simulink model "fulltry"  (R2023b)
settings: Solver=VariableStepAuto  StartTime=0.0  StopTime=40  RelTol=1e-3
undefined symbols (not defined in the file): C_dc, c_drt, C_p_opt, H_gen, H_vsm, H_WTR, I_dc_0, I_dc_base, Ibase_lv, k_d_vsm, k_drt, k_p_p_vsm, k_p_q_vsm, K_pitch, ki_q, L_d, l_f, L_grid, L_q, lambda_opt, Lbase1v, omega_nom, omega_WTR_min, omega_WTR_n, omega_WTR_sl, phase_shift_test_state, phase_shifts, pitch_max, pitch_min, Pitchanglevector, Pmax, Powercoefficient, psi_pm, R_a, r_f, R_grid, R_WTR, rate_max, rate_min, rocof_slope, Rocof_test_state, Sbase1, T_base, T_pitch, T_servo, Tchange_gfm_ref, Trocof_end, Trocof_start, Ts, TSRvector, V_dc, V_dc_base, v_w_n, Vbase_lv, voltage_sag_test_state, wind_array_step, Zbase1v
libraries: spsControlledVoltageSourceLib x6, spsPower3phInstantaneousLib x4, slpidlib x3, spsThreePhaseVIMeasurementLib x3, spsRMSLib x3, spsdq0toabcLib x2, spsCurrentMeasurementLib x2, spsSeriesRLCBranchLib x2, spsVoltageMeasurementLib x2, spsThreePhaseSeriesRLCBranchLib x2, spsDCVoltageSourceLib x2, spsGroundLib x1
(part 1 of 2)
settings Model: Creator=s183702  LastModifiedBy=marti

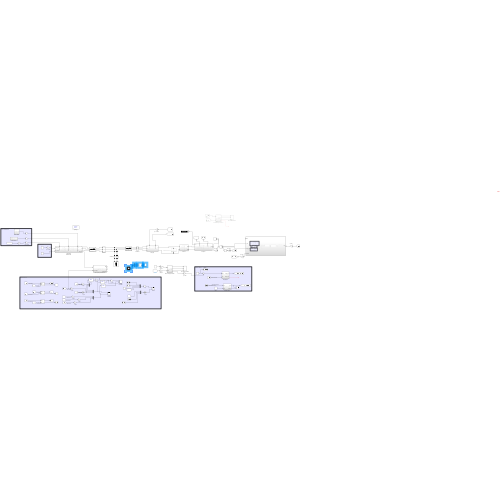
[thumbnail: Simulink's stored preview of the top-level diagram]
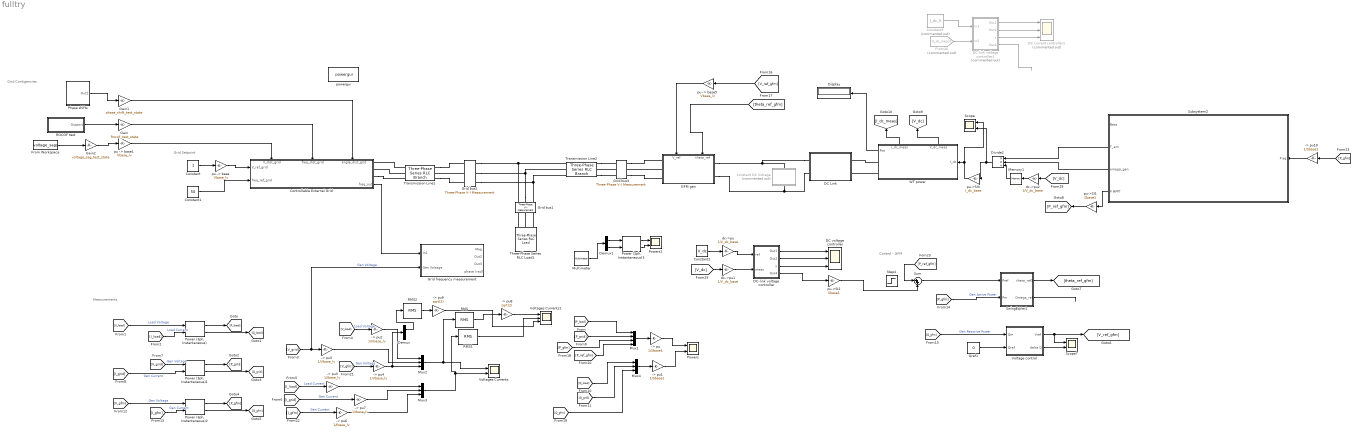
== system fulltry ==
  note: Control - GFM
  note: Grid Setpoint
  note: Grid Contigencies
  note: Measurements
  -> pu : Gain  Gain=1/Sbase1
  -> pu1 : Gain  Gain=1/Sbase1
  -> pu10 : Gain  Gain=1/Sbase1
  -> pu2 : Gain  Gain=1/Vbase_lv
  -> pu3 : Gain  Gain=1/Ibase_lv
  -> pu4 : Gain  Gain=1/Vbase_lv
  -> pu5 : Gain  Gain=1/Vbase_lv
  -> pu6 : Gain  Gain=1/Ibase_lv
  -> pu7 : Gain  Gain=1/Ibase_lv
  -> pu8 : Gain  Gain=sqrt(2)
  -> pu9 : Gain  Gain=sqrt(2)
  Constant : Constant
  Constant1 : Constant  Value=50
  Constant2 : Constant  Value=V_dc
  Constant3 : Constant  Commented=on  Value=I_dc_0
  Controllable External Grid : Subsystem
      settings: PortSchema="{\"entries\":[{\"content\":{\"sides\":[{\"content\":{\"connectorIds\":[\"In1\",\"In2\"]},\"type\":\"ConnectorPlacement.EquallySpacedRectSide\",\"uuid\":\"c82e3ee4-47de-4631-9682-a189e406d2fd\"},{\"content\":{\"connectorIds\":[\"RConn1\",\"RConn2\",\"RConn3\",\"Out1\"],\"side\":\"RIGHT\"},\"type\":\"ConnectorPlacement.EquallySpacedRectSide\",\"uuid\":\"b806e225-811d-4112-8c3d-45e9b8086e84\"},{\"content\":{\"connectorIds\":[\"In3\",\"In4\",\"In5\"],\"side\":\"TOP\"},\"type\":\"ConnectorPlacement.EquallySpacedRectSide\",\"uuid\":\"c79b677b-bc74-4454-b0f0-10f0f27e0767\"}]},\"type\":\"ConnectorPlacement.EquallySpacedConnector\",\"uuid\":\"44354c03-b4f0-403a-803b-b669dc1296a6\"}],\"packageUris\":[\"http://schema.mathworks.com/mf0/Connector/R2020b\"],\"version\":\"1.0\"}"
  DC Link : Subsystem
  DC current controller1 : Scope  Commented=on  NumInputPorts=3
  DC voltage controller : Scope  NumInputPorts=3
  DC-link voltage controller : Subsystem
  DC-link voltage controller1 : Subsystem  Commented=on
  Demux : Demux  Outputs=3
  Demux1 : Demux  Outputs=2
  Display : Display
  Divide2 : Product  Inputs=**/
  From Workspace : FromWorkspace  VariableName=voltage_sags
  From26 : From  Commented=on  GotoTag=I_dc_meas
  GFM gen : Subsystem
      settings: PortSchema="{\"entries\":[{\"content\":{\"sides\":[{\"content\":{\"connectorIds\":[\"LConn1\",\"LConn2\"]},\"type\":\"ConnectorPlacement.EquallySpacedRectSide\",\"uuid\":\"b9b898d8-aa2c-4fc0-879f-33950e845205\"},{\"content\":{\"connectorIds\":[\"RConn1\",\"RConn2\",\"RConn3\"],\"side\":\"RIGHT\"},\"type\":\"ConnectorPlacement.EquallySpacedRectSide\",\"uuid\":\"0f5f2870-ceda-40eb-961f-274893a00dd5\"},{\"content\":{\"connectorIds\":[\"In1\",\"In2\"],\"side\":\"TOP\"},\"type\":\"ConnectorPlacement.EquallySpacedRectSide\",\"uuid\":\"16b0f3cd-2bcf-4c98-bcc9-1e9131637ccf\"}]},\"type\":\"ConnectorPlacement.EquallySpacedConnector\",\"uuid\":\"5f5ec50b-7fca-4ced-b434-e49ba9676af4\"}],\"packageUris\":[\"http://schema.mathworks.com/mf0/Connector/R2020b\"],\"version\":\"1.0\"}"
  Gain : Gain  Gain=Rocof_test_state
  Gain1 : Gain  Gain=phase_shift_test_state
  Gain2 : Gain  Gain=voltage_sag_test_state
  Grid bus1 : spsThreePhaseVIMeasurementLib/Three-Phase V-I Measurement  VoltageMeasurement=phase-to-ground  SetLabelV=on  LabelV=V_load  Vpu=off  VpuLL=off  CurrentMeasurement=yes  SetLabelI=on  LabelI=I_load  Ipu=off  Pbase=100e6  Vbase=500e3  OutputType=Complex  PhasorSimulation=off  PSBequivalent=0
  Grid bus2 : spsThreePhaseVIMeasurementLib/Three-Phase V-I Measurement  VoltageMeasurement=phase-to-ground  SetLabelV=on  LabelV=V_grid  Vpu=off  VpuLL=off  CurrentMeasurement=yes  SetLabelI=on  LabelI=I_grid  Ipu=off  Pbase=100e6  Vbase=500e3  OutputType=Complex  PhasorSimulation=off  PSBequivalent=0
  Grid bus3 : spsThreePhaseVIMeasurementLib/Three-Phase V-I Measurement  VoltageMeasurement=phase-to-ground  SetLabelV=on  LabelV=V_gfm  Vpu=off  VpuLL=off  CurrentMeasurement=yes  SetLabelI=on  LabelI=I_gfm  Ipu=off  Pbase=100e6  Vbase=500e3  OutputType=Complex  PhasorSimulation=off  PSBequivalent=0
  Grid frequency measurement : Subsystem
  Memory1 : Memory  InitialCondition=V_dc
  Multimeter : spsMultimeterLib/Multimeter  L=6  sel=[1 2 3 4 5 6]  yselected={}  Gain=[1 1 1 1 1 1]  OutputType=Complex  PlotAtSimulationStop=off  PhasorSimulation=off
  Mux1 : Mux
  Mux2 : Mux  Inputs=3
  Mux3 : Mux  Inputs=3
  Mux4 : Mux  Inputs=3
  Phase shifts : Subsystem
  Power (3ph, Instantaneous){,1..3} (4 alike) : spsPower3phInstantaneousLib/Power (3ph, Instantaneous)
  Powers : Scope  NumInputPorts=2
  Powers1 : Scope  NumInputPorts=2
  Qref1 : Constant  Value=0
  RMS : spsRMSLib/RMS  TrueRMS=off  Freq=50  RMSInit=1  Ts=0
  RMS1 : spsRMSLib/RMS  TrueRMS=off  Freq=50  RMSInit=1  Ts=0
  RMS2 : spsRMSLib/RMS  TrueRMS=off  Freq=50  RMSInit=1  Ts=0
  ROCOF test : Subsystem
  Scope : Scope  NumInputPorts=2
  Scope7 : Scope  NumInputPorts=2
  Step4 : Step  Time=Tchange_gfm_ref  Before=Sbase1  After=Sbase1  SampleTime=0
  Subsystem2 : Subsystem
  Sum : Sum  Inputs=|++
  SwingEqVer1 : Subsystem
  Three-Phase Series RLC Load1 : spsThreePhaseSeriesRLCLoadLib/Three-Phase Series RLC Load  LConnTagsString=A|B|C  Configuration=Y (grounded)  NominalVoltage=Vbase_lv*sqrt(3/2)  Vabc=[1e3 1e3 1e3]  Vabcp=[1e3 1e3 1e3]  NominalFrequency=f_nom  UnbalancedPower=off  ActivePower=Sbase1*0.2  InductivePower=0  CapacitivePower=0  Pabc=[10e3 9e3 11e3]  QLabc=[100 90 110]  QCabc=[100 90 110]  Pabcp=[10e3 9e3 11e3]  QLabcp=[100 90 110]  QCabcp=[100 90 110]  Measurements=Branch voltages and currents  LoadType=constant PQ
  Transmission Line1 : spsThreePhaseSeriesRLCBranchLib/Three-Phase Series RLC Branch  LConnTagsString=A|B|C  RConnTagsString=A|B|C  BranchType=RL  Resistance=R_grid  Inductance=L_grid  Capacitance=0  Measurements=None
  Transmission Line2 : spsThreePhaseSeriesRLCBranchLib/Three-Phase Series RLC Branch  LConnTagsString=A|B|C  RConnTagsString=A|B|C  BranchType=RL  Resistance=r_f*Zbase1v  Inductance=l_f*Lbase1v  Capacitance=0  Measurements=None
  Voltage control : Subsystem
  Voltages Currents : Scope  NumInputPorts=2
  Voltages Currents1 : Scope  NumInputPorts=3
  WT power : Subsystem
      settings: PortSchema="{\"entries\":[{\"content\":{\"sides\":[{\"content\":{\"connectorIds\":[\"In1\"]},\"type\":\"ConnectorPlacement.EquallySpacedRectSide\",\"uuid\":\"9d3e38d2-6add-483d-9a31-3b5598dff8d3\"},{\"content\":{\"connectorIds\":[\"Out1\",\"RConn1\",\"RConn2\"],\"side\":\"RIGHT\"},\"type\":\"ConnectorPlacement.EquallySpacedRectSide\",\"uuid\":\"7ce5d226-07b0-4d85-bacd-eba224635451\"},{\"content\":{\"connectorIds\":[\"Out2\",\"Out3\"],\"side\":\"TOP\"},\"type\":\"ConnectorPlacement.EquallySpacedRectSide\",\"uuid\":\"1864accd-580c-4e01-b41e-4bc1921d0b77\"},{\"content\":{\"side\":\"BOTTOM\"},\"type\":\"ConnectorPlacement.EquallySpacedRectSide\",\"uuid\":\"0a771f6d-f5fb-412d-b2d7-9d95c39f39de\"}]},\"type\":\"ConnectorPlacement.EquallySpacedConnector\",\"uuid\":\"874bd654-abb7-47d1-80fe-1eaf36f4fe8a\"}],\"packageUris\":[\"http://schema.mathworks.com/mf0/Connector/R2020b\"],\"version\":\"1.0\"}"
  constant DC Voltage : Subsystem  Commented=on
  dc->pu : Gain  Gain=1/V_dc_base
  dc->pu1 : Gain  Gain=1/V_dc_base
  dc->pu2 : Gain  Gain=1/V_dc_base
  powergui : sps_lib/powergui  Priority=1  SimulationMode=Discrete  SampleTime=Ts  frequency=60  Iterations=50  frequencyindice=0  Pbase=100e6  ErrMax=1e-4  UnitsV=kV  UnitsW=MW  buscounter=0  FunctionMessages=off  echomessages=off  EnableUseOfTLC=off  CurrentSourceSwitches=off  DisableSnubberDevices=off  DisableRonSwitches=off  DisableVfSwitches=off  DisplayEquations=off  AutomaticDiscreteSolvers=off  SolverType=Tustin/Backward Euler (TBE)  Interpol=off  ExternalGateDelay=off  methode=off  Ts=100  x0status=blocks  SPID=on  SwTol=0  HookPort=off  NonlinearTolerance=1e-4  nMaxIteration=100  ContinueOnMaxIteration=off  RestoreLinks=warning  ResistiveCurrentMeasurement=off  Frange=[0:2:500]  Ylog=off  Xlog=on  ShowGrid=off  save=off  variable=ZData  structure=0  ZoomFFT=off  StartTime=0.0  cycles=1  DisplayStyle=1  fundamental=60  FreqAxis=off  MaxFrequency=1000  frequencyindicesteady=1  RmsSteady=1  display=off
  "pu -> base" : Gain  Gain=Vbase_lv
  "pu -> base1" : Gain  Gain=Vbase_lv
  "pu -> base5" : Gain  Gain=Vbase_lv
  pu->SI1 : Gain  Gain=Sbase1
  pu->SI2 : Gain  Gain=Sbase1
  pu->SI3 : Gain  Gain=I_dc_base
  wires:
  SwingEqVer1/2(Omega_ref) -> ?
  -> pu3/1 -> Mux3/1
  "Power (3ph, Instantaneous)"/1 -> [P_load]
  Mux3/1 -> RMS1/1, Voltages Currents/2
  Qref1/1 -> Voltage control/2(Qref)
  RMS1/1 -> Voltages Currents1/2
  RMS/1 -> -> pu8/1
  -> pu9/1 -> Voltages Currents1/3
  -> pu8/1 -> Voltages Currents1/1
  WT power/1(Pwt) -> Display/1
  From Workspace/1 -> Gain2/1
  [V_gfm] -> -> pu4/1  "Gen Voltage"
  RMS2/1 -> -> pu9/1
  Constant3/1 -> DC-link voltage controller1/1(In1)
  Phase shifts/1(Out2) -> Gain1/1
  dc->pu/1 -> DC-link voltage controller/1(ref)
  Gain/1 -> Controllable External Grid/4(freq_dist_grid)
  From26/1 -> DC-link voltage controller1/2(In2)
  -> pu4/1 -> Demux/1, Mux2/3
  -> pu1/1 -> Powers/2
  Controllable External Grid/1(freq_out) -> Grid frequency measurement/1(In1)
  Gain1/1 -> Controllable External Grid/5(angle_dist_grid)
  DC-link voltage controller/3(y) -> DC voltage controller/3
  [V_ref_gfm] -> "pu -> base5"/1
  Demux/1 -> RMS2/1
  pu->SI2/1 -> Sum/2
  [P_ref_gfm] -> Sum/1
  DC-link voltage controller1/2(Out2) -> DC current controller1/2
  [V_gfm] -> "Power (3ph, Instantaneous)2"/1  "Gen Voltage"
  DC-link voltage controller/4(Out4) -> pu->SI2/1
  WT power/3(i_dc_meas) -> [I_dc_meas]
  Mux4/1 -> -> pu1/1
  dc->pu1/1 -> DC-link voltage controller/2(meas)
  DC-link voltage controller1/3(y) -> DC current controller1/3
  [Q_gfm] -> Voltage control/1(Qm)  "Gen Reactive Power"
  Divide2/1 -> Scope/2, pu->SI3/1
  Constant2/1 -> dc->pu/1
  Memory1/1 -> Divide2/3
  Subsystem2/2(T_em) -> Divide2/1
  "Power (3ph, Instantaneous)"/2 -> [Q_load]
  [Q_load] -> Mux4/1
  DC-link voltage controller1/1(Out1) -> DC current controller1/1
  [Q_grid] -> Mux4/2
  -> pu5/1 -> Mux2/2
  "Power (3ph, Instantaneous)1"/1 -> [P_grid]
  DC-link voltage controller/1(Out1) -> DC voltage controller/1
  DC-link voltage controller/2(Out2) -> DC voltage controller/2
  WT power/2(V_dc_meas) -> [V_dc]
  [V_dc] -> dc->pu1/1
  [P_gfm] -> Mux1/3
  Voltage control/1(Vref) -> Scope7/1, [V_ref_gfm]
  [V_grid] -> Grid frequency measurement/2(Gen Voltage), -> pu5/1  "Gen Voltage"
  -> pu2/1 -> Mux2/1
  Voltage control/2(delta Q) -> Scope7/2
  [P_ref_gfm] -> Mux1/4
  DC-link voltage controller1/4(Out4) -> ?
  [I_load] -> "Power (3ph, Instantaneous)"/2  "Load Current"
  Mux1/1 -> -> pu/1
  -> pu/1 -> Powers/1
  [P_load] -> Mux1/1
  [P_grid] -> Mux1/2
  Mux2/1 -> RMS/1, Voltages Currents/1
  Gain2/1 -> "pu -> base1"/1
  [theta_ref_gfm] -> GFM gen/1(theta_ref)
  [I_gfm] -> "Power (3ph, Instantaneous)2"/2  "Gen Current"
  [I_gfm] -> -> pu6/1  "Gen Current"
  [V_grid] -> "Power (3ph, Instantaneous)1"/1  "Gen Voltage"
  [V_load] -> -> pu2/1  "Load Voltage"
  "Power (3ph, Instantaneous)1"/2 -> [Q_grid]
  "pu -> base"/1 -> Controllable External Grid/1(V_ref_grid)
  [V_load] -> "Power (3ph, Instantaneous)"/1  "Load Voltage"
  [I_grid] -> -> pu7/1  "Gen Current"
  [I_load] -> -> pu3/1  "Load Current"
  [Q_gfm] -> Mux4/3
  [I_grid] -> "Power (3ph, Instantaneous)1"/2  "Gen Current"
  "pu -> base5"/1 -> GFM gen/2(V_ref)
  Constant1/1 -> Controllable External Grid/2(freq_ref_grid)
  Constant/1 -> "pu -> base"/1
  -> pu6/1 -> Mux3/3
  "Power (3ph, Instantaneous)2"/2 -> [Q_gfm]
  Sum/1 -> SwingEqVer1/1(Pref)
  ROCOF test/1(Outport) -> Gain/1
  "pu -> base1"/1 -> Controllable External Grid/3(V_dist_grid)
  SwingEqVer1/1(theta_ref1) -> [theta_ref_gfm]
  "Power (3ph, Instantaneous)2"/1 -> [P_gfm]
  [P_gfm] -> SwingEqVer1/2(Pm)  "Gen Active Power"
  -> pu7/1 -> Mux3/2
  ? -> ?
  Subsystem2/3(omega_gen) -> Divide2/2
  Subsystem2/4(P MPPT) -> pu->SI1/1
  -> pu10/1 -> Subsystem2/1(P ag)
  [P_gfm] -> -> pu10/1
  pu->SI1/1 -> [P_ref_gfm]
  [V_dc] -> dc->pu2/1
  dc->pu2/1 -> Memory1/1
  pu->SI3/1 -> Scope/1, WT power/1(I_dc)
  Multimeter/1 -> Demux1/1
  Demux1/1 -> "Power (3ph, Instantaneous)3"/1
  Demux1/2 -> "Power (3ph, Instantaneous)3"/2
  "Power (3ph, Instantaneous)3"/1 -> Powers1/1
  "Power (3ph, Instantaneous)3"/2 -> Powers1/2
  connections:
  DC Link/LConn2 -- GFM gen/LConn2 -- constant DC Voltage/RConn1
  DC Link/LConn1 -- GFM gen/LConn1 -- constant DC Voltage/LConn1
  Grid bus2/RConn1 -- Grid bus1/LConn1 -- Transmission Line2/LConn1
  Grid bus2/RConn3 -- Grid bus1/LConn3 -- Transmission Line2/LConn3
  Grid bus1/LConn2 -- Transmission Line2/LConn2 -- Grid bus2/RConn2
  WT power/RConn1 -- DC Link/RConn1
  Grid bus2/LConn2 -- Transmission Line1/RConn2
  Grid bus3/LConn1 -- GFM gen/RConn1
  Three-Phase Series RLC Load1/LConn3 -- Grid bus1/RConn3
  Transmission Line2/RConn1 -- Grid bus3/RConn1
  Controllable External Grid/RConn3 -- Transmission Line1/LConn3
  GFM gen/RConn2 -- Grid bus3/LConn2
  Transmission Line1/LConn1 -- Controllable External Grid/RConn1
  Three-Phase Series RLC Load1/LConn1 -- Grid bus1/RConn1
  Transmission Line1/RConn1 -- Grid bus2/LConn1
  Transmission Line1/RConn3 -- Grid bus2/LConn3
  Three-Phase Series RLC Load1/LConn2 -- Grid bus1/RConn2
  Transmission Line1/LConn2 -- Controllable External Grid/RConn2
  Grid bus3/LConn3 -- GFM gen/RConn3
  Grid bus3/RConn2 -- Transmission Line2/RConn2
  Transmission Line2/RConn3 -- Grid bus3/RConn3
  WT power/RConn2 -- DC Link/RConn2

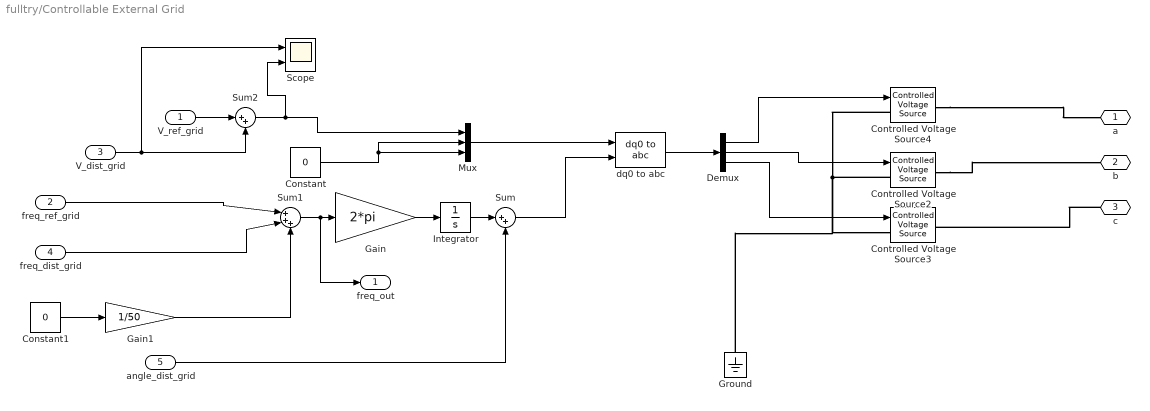
== system fulltry/Controllable External Grid ==
  V_ref_grid : Inport
  freq_ref_grid : Inport  Port=2
  V_dist_grid : Inport  Port=3
  freq_dist_grid : Inport  Port=4
  angle_dist_grid : Inport  Port=5
  Constant : Constant  Value=0
  Constant1 : Constant  Value=0
  Controlled Voltage Source2 : spsControlledVoltageSourceLib/Controlled Voltage Source  Initialize=on  Source_Type=AC  Amplitude=Vbase_lv  Phase=-120  Frequency=50  Measurements=None
  Controlled Voltage Source3 : spsControlledVoltageSourceLib/Controlled Voltage Source  Initialize=on  Source_Type=AC  Amplitude=Vbase_lv  Phase=120  Frequency=50  Measurements=None
  Controlled Voltage Source4 : spsControlledVoltageSourceLib/Controlled Voltage Source  Initialize=on  Source_Type=AC  Amplitude=Vbase_lv  Phase=0  Frequency=50  Measurements=None
  Demux : Demux  Outputs=3
  Gain : Gain  Gain=2*pi
  Gain1 : Gain  Gain=1/50
  Ground : spsGroundLib/Ground  LConnTagsString=a
  Integrator : Integrator
  Mux : Mux  Inputs=3
  Scope : Scope  NumInputPorts=2
  Sum : Sum  Inputs=|++
  Sum1 : Sum  Inputs=|+++
  Sum2 : Sum  Inputs=|++
  dq0 to abc : spsdq0toabcLib/dq0 to abc  Alignment=Aligned with phase A axis
  a : PMIOPort  Side=Right
  b : PMIOPort  Port=2  Side=Right
  c : PMIOPort  Port=3  Side=Right
  freq_out : Outport
  wires:
  Demux/1 -> Controlled Voltage Source4/1
  Demux/2 -> Controlled Voltage Source2/1
  Demux/3 -> Controlled Voltage Source3/1
  Mux/1 -> dq0 to abc/1
  Constant/1 -> Mux/2, Mux/3
  dq0 to abc/1 -> Demux/1
  Sum2/1 -> Scope/2, Mux/1
  Gain/1 -> Integrator/1
  Integrator/1 -> Sum/1
  angle_dist_grid/1 -> Sum/2
  freq_dist_grid/1 -> Sum1/2
  Sum1/1 -> freq_out/1, Gain/1
  freq_ref_grid/1 -> Sum1/1
  Sum/1 -> dq0 to abc/2
  V_ref_grid/1 -> Sum2/1
  V_dist_grid/1 -> Sum2/2, Scope/1
  Gain1/1 -> Sum1/3
  Constant1/1 -> Gain1/1
  connections:
  Controlled Voltage Source2/LConn1 -- Controlled Voltage Source4/LConn1 -- Ground/LConn1 -- Controlled Voltage Source3/LConn1
  c/RConn1 -- Controlled Voltage Source3/RConn1
  Controlled Voltage Source4/RConn1 -- a/RConn1
  Controlled Voltage Source2/RConn1 -- b/RConn1

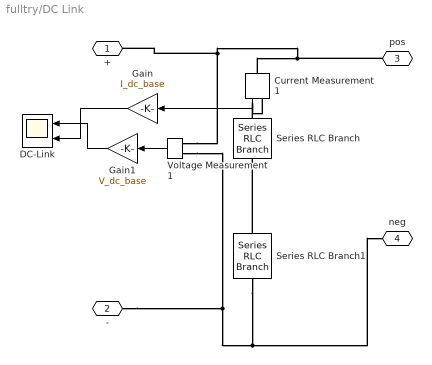
== system fulltry/DC Link ==
  Current Measurement1 : spsCurrentMeasurementLib/Current Measurement  PhasorSimulation=off  OutputType=Complex  PSBequivalent=0
  DC-Link : Scope  NumInputPorts=2
  Gain : Gain  Gain=I_dc_base
  Gain1 : Gain  Gain=V_dc_base
  Series RLC Branch : spsSeriesRLCBranchLib/Series RLC Branch  LConnTagsString=__new0  RConnTagsString=__new0  BranchType=C  Resistance=1  Inductance=1e-3  SetiL0=off  InitialCurrent=0  Capacitance=C_dc/2  Setx0=on  InitialVoltage=V_dc/2  Measurements=None
  Series RLC Branch1 : spsSeriesRLCBranchLib/Series RLC Branch  LConnTagsString=__new0  RConnTagsString=__new0  BranchType=C  Resistance=1  Inductance=1e-3  SetiL0=off  InitialCurrent=0  Capacitance=C_dc/2  Setx0=on  InitialVoltage=V_dc/2  Measurements=None
  Voltage Measurement1 : spsVoltageMeasurementLib/Voltage Measurement  PhasorSimulation=off  OutputType=Complex  PSBequivalent=0
  + : PMIOPort  Side=Left
  - : PMIOPort  Port=2  Side=Left
  pos : PMIOPort  Port=3  Side=Right
  neg : PMIOPort  Port=4  Side=Right
  wires:
  Voltage Measurement1/1 -> Gain1/1
  Current Measurement1/1 -> Gain/1
  Gain/1 -> DC-Link/2
  Gain1/1 -> DC-Link/1
  connections:
  -/RConn1 -- Series RLC Branch1/RConn1 -- neg/RConn1 -- Voltage Measurement1/LConn2
  Series RLC Branch1/LConn1 -- Series RLC Branch/RConn1
  pos/RConn1 -- Current Measurement1/LConn1 -- +/RConn1 -- Voltage Measurement1/LConn1
  Series RLC Branch/LConn1 -- Current Measurement1/RConn1

== system fulltry/DC-link voltage controller ==
  ref : Inport
  meas : Inport  Port=2
  Gain : Gain  Gain=-1
  Mux : Mux  Inputs=2
  PID Controller : slpidlib/PID Controller  Controller=PI  Form=Parallel  TimeDomain=Continuous-time  UseExternalTs=off  SampleTime=-1  IntegratorMethod=Forward Euler  FilterMethod=Forward Euler  ControllerParametersSource=internal  P=5  I=1  UseKiTs=off  D=0  N=100  UseFilter=on  TunerSelectOption=Transfer Function Based (PID Tuner App)  InitialConditionSource=internal  InitialConditionForIntegrator=0  InitialConditionForFilter=0  DifferentiatorICPrevScaledInput=0  ExternalReset=none  TrackingMode=off  Kt=1  LimitOutput=off  SatLimitsSource=internal  UpperSaturationLimit=inf  LowerSaturationLimit=-inf  LinearizeAsGain=on  AntiWindupMode=none  Kb=1  LimitIntegrator=off  UpperIntegratorSaturationLimit=inf  LowerIntegratorSaturationLimit=-inf  POutMin=[]  POutMax=[]  IOutMin=[]  IOutMax=[]  DOutMin=[]  DOutMax=[]  NOutMin=[]  NOutMax=[]  SumOutMin=[]  SumOutMax=[]  SaturationOutMin=[]  SaturationOutMax=[]  PParamMin=[]  PParamMax=[]  IParamMin=[]  IParamMax=[]  DParamMin=[]  DParamMax=[]  NParamMin=[]  NParamMax=[]  KbParamMin=[]  KbParamMax=[]  KtParamMin=[]  KtParamMax=[]  KbOutMin=[]  KbOutMax=[]  KtOutMin=[]  KtOutMax=[]  IntegratorOutMin=[]  IntegratorOutMax=[]  FilterOutMin=[]  FilterOutMax=[]  SumI1OutMin=[]  SumI1OutMax=[]  SumI2OutMin=[]  SumI2OutMax=[]  SumI3OutMin=[]  SumI3OutMax=[]  SumI4OutMin=[]  SumI4OutMax=[]  SumDOutMin=[]  SumDOutMax=[]  DifferentiatorOutMin=[]  DifferentiatorOutMax=[]  FilterDiffOutCoefMin=[]  FilterDiffOutCoefMax=[]  ReciprocalOutMin=[]  ReciprocalOutMax=[]  SumDenOutMin=[]  SumDenOutMax=[]  SumNumOutMin=[]  SumNumOutMax=[]  DivideOutMin=[]  DivideOutMax=[]  UdiffTsProdOutMin=[]  UdiffTsProdOutMax=[]  NTsProdOutMin=[]  NTsProdOutMax=[]  UintegralTsProdOutMin=[]  UintegralTsProdOutMax=[]  UngainTsProdOutMin=[]  UngainTsProdOutMax=[]  ClampingZeroOutDataTypeStr=Inherit: Inherit via back propagation  ClampingZeroOutMin=[]  ClampingZeroOutMax=[]  FilterDenConstantOutDataTypeStr=Inherit: Inherit via back propagation  FilterDenConstantOutMin=[]  FilterDenConstantOutMax=[]  PCopyOutDataTypeStr=Inherit: Inherit via back propagation  PCopyOutMin=[]  PCopyOutMax=[]  NCopyOutDataTypeStr=Inherit: Inherit via back propagation  NCopyOutMin=[]  NCopyOutMax=[]  IntegratorContinuousStateAttributes=''  IntegratorStateMustResolveToSignalObject=off  IntegratorRTWStateStorageClass=Auto  FilterContinuousStateAttributes=''  FilterStateMustResolveToSignalObject=off  FilterRTWStateStorageClass=Auto  ParallelPVariant=InternalParameters  IdealPVariant=Disabled  IVariant=InternalParameters  DVariant=Disabled  IntegratorVariant=Continuous  SatVariant=Disabled  AWVariant=Passthrough  PCopyVariant=Disabled  TRVariant=Disabled  FdbkBlocksVariant=Forward  IdealPFdbkVariant=Disabled  SatFdbkVariant=Disabled  DerivativeFilterVariant=Disabled  NVariant=Disabled  NCopyVariant=Disabled_SignalSpec  FilterICVariant=Disabled  IntegratorICVariant=InternalICs  ExternalResetVariant=Disabled  TRSumVariant=Passthrough  SumFdbkVariant=Disabled  SumVariant=Sum_PI  TsampFilterVariant=InternalTs  TsampNgainVariant=Passthrough  TsampIntegralVariant=Disabled_SignalSpec  ExternalSaturationOutDataTypeStr=Inherit: Same as second input
  Sum : Sum  Inputs=+-|
  Out1 : Outport
  Out2 : Outport  Port=2
  y : Outport  Port=3
  Out4 : Outport  Port=4
  wires:
  Sum/1 -> Out2/1, PID Controller/1
  meas/1 -> Mux/2, Sum/2
  ref/1 -> Mux/1, Sum/1
  Mux/1 -> Out1/1
  PID Controller/1 -> y/1, Gain/1
  Gain/1 -> Out4/1

== system fulltry/DC-link voltage controller1 ==
  In1 : Inport
  In2 : Inport  Port=2
  Gain : Gain  Commented=through  Gain=Sbase1
  Gain1 : Gain  Gain=1/I_dc_base
  Mux : Mux  Inputs=2
  PID Controller : slpidlib/PID Controller  Controller=PI  Form=Parallel  TimeDomain=Continuous-time  UseExternalTs=off  SampleTime=-1  IntegratorMethod=Forward Euler  FilterMethod=Forward Euler  ControllerParametersSource=internal  P=0.1  I=0  UseKiTs=off  D=0  N=100  UseFilter=on  TunerSelectOption=Transfer Function Based (PID Tuner App)  InitialConditionSource=internal  InitialConditionForIntegrator=1  InitialConditionForFilter=0  DifferentiatorICPrevScaledInput=0  ExternalReset=none  TrackingMode=off  Kt=1  LimitOutput=off  SatLimitsSource=internal  UpperSaturationLimit=inf  LowerSaturationLimit=-inf  LinearizeAsGain=on  AntiWindupMode=none  Kb=1  LimitIntegrator=off  UpperIntegratorSaturationLimit=inf  LowerIntegratorSaturationLimit=-inf  POutMin=[]  POutMax=[]  IOutMin=[]  IOutMax=[]  DOutMin=[]  DOutMax=[]  NOutMin=[]  NOutMax=[]  SumOutMin=[]  SumOutMax=[]  SaturationOutMin=[]  SaturationOutMax=[]  PParamMin=[]  PParamMax=[]  IParamMin=[]  IParamMax=[]  DParamMin=[]  DParamMax=[]  NParamMin=[]  NParamMax=[]  KbParamMin=[]  KbParamMax=[]  KtParamMin=[]  KtParamMax=[]  KbOutMin=[]  KbOutMax=[]  KtOutMin=[]  KtOutMax=[]  IntegratorOutMin=[]  IntegratorOutMax=[]  FilterOutMin=[]  FilterOutMax=[]  SumI1OutMin=[]  SumI1OutMax=[]  SumI2OutMin=[]  SumI2OutMax=[]  SumI3OutMin=[]  SumI3OutMax=[]  SumI4OutMin=[]  SumI4OutMax=[]  SumDOutMin=[]  SumDOutMax=[]  DifferentiatorOutMin=[]  DifferentiatorOutMax=[]  FilterDiffOutCoefMin=[]  FilterDiffOutCoefMax=[]  ReciprocalOutMin=[]  ReciprocalOutMax=[]  SumDenOutMin=[]  SumDenOutMax=[]  SumNumOutMin=[]  SumNumOutMax=[]  DivideOutMin=[]  DivideOutMax=[]  UdiffTsProdOutMin=[]  UdiffTsProdOutMax=[]  NTsProdOutMin=[]  NTsProdOutMax=[]  UintegralTsProdOutMin=[]  UintegralTsProdOutMax=[]  UngainTsProdOutMin=[]  UngainTsProdOutMax=[]  ClampingZeroOutDataTypeStr=Inherit: Inherit via back propagation  ClampingZeroOutMin=[]  ClampingZeroOutMax=[]  FilterDenConstantOutDataTypeStr=Inherit: Inherit via back propagation  FilterDenConstantOutMin=[]  FilterDenConstantOutMax=[]  PCopyOutDataTypeStr=Inherit: Inherit via back propagation  PCopyOutMin=[]  PCopyOutMax=[]  NCopyOutDataTypeStr=Inherit: Inherit via back propagation  NCopyOutMin=[]  NCopyOutMax=[]  IntegratorContinuousStateAttributes=''  IntegratorStateMustResolveToSignalObject=off  IntegratorRTWStateStorageClass=Auto  FilterContinuousStateAttributes=''  FilterStateMustResolveToSignalObject=off  FilterRTWStateStorageClass=Auto  ParallelPVariant=InternalParameters  IdealPVariant=Disabled  IVariant=InternalParameters  DVariant=Disabled  IntegratorVariant=Continuous  SatVariant=Disabled  AWVariant=Passthrough  PCopyVariant=Disabled  TRVariant=Disabled  FdbkBlocksVariant=Forward  IdealPFdbkVariant=Disabled  SatFdbkVariant=Disabled  DerivativeFilterVariant=Disabled  NVariant=Disabled  NCopyVariant=Disabled_SignalSpec  FilterICVariant=Disabled  IntegratorICVariant=InternalICs  ExternalResetVariant=Disabled  TRSumVariant=Passthrough  SumFdbkVariant=Disabled  SumVariant=Sum_PI  TsampFilterVariant=InternalTs  TsampNgainVariant=Passthrough  TsampIntegralVariant=Disabled_SignalSpec  ExternalSaturationOutDataTypeStr=Inherit: Same as second input
  Sum : Sum  Inputs=+-|
  Out1 : Outport
  Out2 : Outport  Port=2
  y : Outport  Port=3
  Out4 : Outport  Port=4
  wires:
  Gain/1 -> Out4/1
  PID Controller/1 -> Gain/1, y/1
  Mux/1 -> Out1/1
  In1/1 -> Sum/1, Mux/1
  In2/1 -> Sum/2, Mux/2
  Sum/1 -> Gain1/1, Out2/1
  Gain1/1 -> PID Controller/1

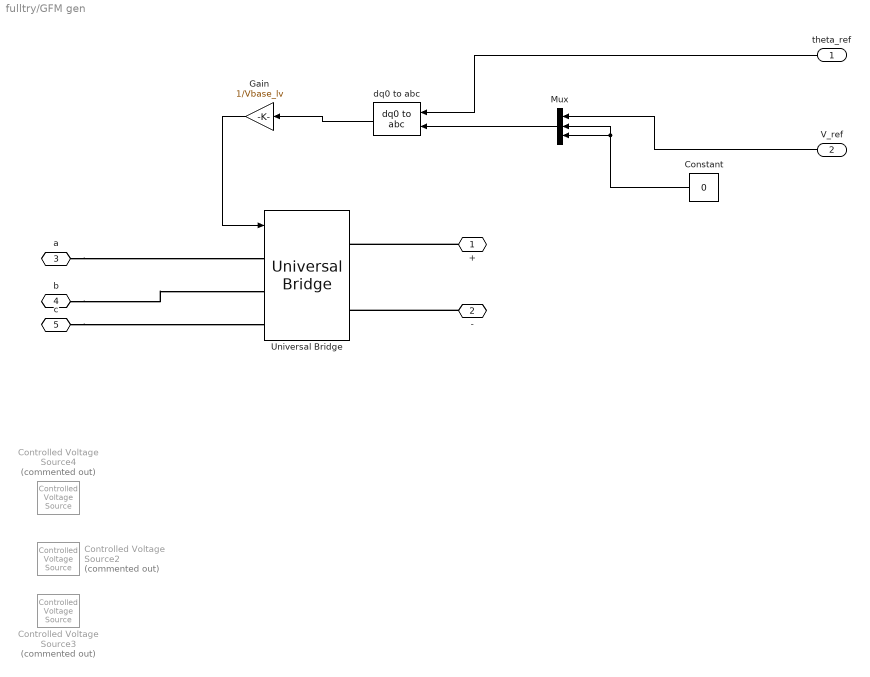
== system fulltry/GFM gen ==
  theta_ref : Inport
  V_ref : Inport  Port=2
  Constant : Constant  Value=0
  Controlled Voltage Source2 : spsControlledVoltageSourceLib/Controlled Voltage Source  Commented=on  Initialize=on  Source_Type=AC  Amplitude=Vbase_lv  Phase=-120  Frequency=50  Measurements=None
  Controlled Voltage Source3 : spsControlledVoltageSourceLib/Controlled Voltage Source  Commented=on  Initialize=on  Source_Type=AC  Amplitude=Vbase_lv  Phase=120  Frequency=50  Measurements=None
  Controlled Voltage Source4 : spsControlledVoltageSourceLib/Controlled Voltage Source  Commented=on  Initialize=on  Source_Type=AC  Amplitude=Vbase_lv  Phase=0  Frequency=50  Measurements=None
  Gain : Gain  Gain=1/Vbase_lv
  Mux : Mux  Inputs=3
  Universal Bridge : spsUniversalBridgeLib/Universal Bridge  Arms=3  SnubberResistance=1e5  SnubberCapacitance=inf  Device=Average-model based VSC  Ron=1e-3  Lon=0  ForwardVoltages="[  0  0  ]"  ForwardVoltage=0  GTOparameters=[ 10e-6 , 20e-6 ]  IGBTparameters=[ 1e-6 , 2e-6 ]  Measurements=None  Measurements_2=None  converterType=Rectifier
  dq0 to abc : spsdq0toabcLib/dq0 to abc  Alignment=Aligned with phase A axis
  + : PMIOPort  Side=Left
  - : PMIOPort  Port=2  Side=Left
  a : PMIOPort  Port=3  Side=Right
  b : PMIOPort  Port=4  Side=Right
  c : PMIOPort  Port=5  Side=Right
  wires:
  Mux/1 -> dq0 to abc/1
  Constant/1 -> Mux/2, Mux/3
  dq0 to abc/1 -> Gain/1
  V_ref/1 -> Mux/1
  theta_ref/1 -> dq0 to abc/2
  Gain/1 -> Universal Bridge/1
  connections:
  c/RConn1 -- Universal Bridge/LConn3
  a/RConn1 -- Universal Bridge/LConn1
  b/RConn1 -- Universal Bridge/LConn2
  -/RConn1 -- Universal Bridge/RConn2
  +/RConn1 -- Universal Bridge/RConn1

== system fulltry/Grid frequency measurement ==
  In1 : Inport
  Gen Voltage : Inport  Port=2
  Demux1 : Demux  Outputs=3
  Fourier : spsFourierLib/Fourier  Freq=50  n=1  InInit=[Vbase_lv, 0]  Ts=0
  Frequency (Phasor) : spsFrequencyPhasorLib/Frequency (Phasor)  Fn=50  T=0.1
      settings: LibrarySourceBlock=|
      | sps_lib/Sensors and Measurements/Frequency
      | (Phasor)
  Scope : Scope  Commented=on  NumInputPorts=2
  Mag : Outport
  Out2 : Outport  Port=2
  Out3 : Outport  Port=3
  "phase (rad) " : Outport  Port=4
  wires:
  Frequency (Phasor)/2 -> "phase (rad) "/1
  Demux1/3 -> Out3/1
  In1/1 -> Scope/1
  Fourier/2 -> Frequency (Phasor)/1
  Demux1/2 -> Out2/1
  Frequency (Phasor)/1 -> Scope/2
  Demux1/1 -> Fourier/1
  Fourier/1 -> Mag/1
  Gen Voltage/1 -> Demux1/1

== system fulltry/Phase shifts ==
  From Workspace : FromWorkspace  Commented=on  VariableName=phase_shifts  OutputAfterFinalValue=Setting to zero
  Step : Step  Time=phase_shifts(1,1)  After=phase_shifts(1,2)  SampleTime=0
  Step1 : Step  Time=phase_shifts(2,1)  After=phase_shifts(2,2)  SampleTime=0
  Step2 : Step  Time=phase_shifts(3,1)  After=phase_shifts(3,2)  SampleTime=0
  Sum1 : Sum  Inputs=+++
  Out2 : Outport
  wires:
  Sum1/1 -> Out2/1
  Step/1 -> Sum1/1
  Step2/1 -> Sum1/3
  From Workspace/1 -> ?
  Step1/1 -> Sum1/2

== system fulltry/ROCOF test ==
  Clock : Clock
  Constant4 : Constant  Value=0
  Constant5 : Constant
  Ramp : simulink/Sources/Ramp  slope=rocof_slope  start=Trocof_start  InitialOutput=0
  Sample and Hold : spsSampleandHoldLib/Sample and Hold  ic=0  Ts=0
      settings: LibrarySourceBlock=|
      | sps_lib/Control/Sample and
      | Hold
  Switch : Switch  Criteria=u2 > Threshold  Threshold=Trocof_start  SaturateOnIntegerOverflow=off  InputSameDT=off
  Switch1 : Switch  Threshold=Trocof_end  SaturateOnIntegerOverflow=off  InputSameDT=off
  Outport : Outport
  wires:
  Clock/1 -> Switch/2, Switch1/2
  Constant4/1 -> Switch/3, Switch1/1
  Sample and Hold/1 -> Outport/1
  Ramp/1 -> Switch/1
  Constant5/1 -> Switch1/3
  Switch/1 -> Sample and Hold/1
  Switch1/1 -> Sample and Hold/2

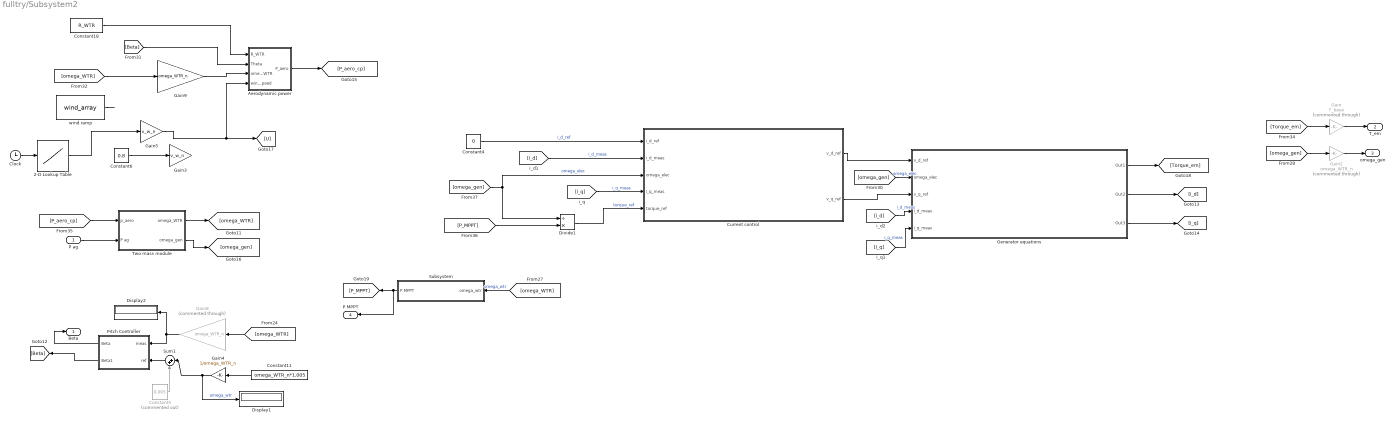
== system fulltry/Subsystem2 ==
  P ag : Inport
  2-D Lookup Table : Lookup_n-D  NumberOfTableDimensions=1  BreakpointsForDimension1=wind_array_step(1,:)  BreakpointsForDimension2=[1:3]  IndexSearchMethod=Linear search  Table=wind_array_step(2,:)  InterpMethod=Nearest  InternalRulePriority=Speed  RndMeth=Simplest
  Aerodynamic power : Subsystem
  Clock : Clock
  Constant11 : Constant  Value=omega_WTR_n*1.005
  Constant18 : Constant  Value=R_WTR
  Constant4 : Constant  Value=0
  Constant5 : Constant  Commented=on  Value=0.005
  Constant6 : Constant  Value=0.8
  Current control : Subsystem
  Display1 : Display
  Display2 : Display
  Divide1 : Product  Inputs=/*
  Gain : Gain  Commented=through  Gain=T_base
  Gain2 : Gain  Commented=through  Gain=omega_WTR_n
  Gain3 : Gain  Gain=v_w_n
  Gain4 : Gain  Gain=1/omega_WTR_n
  Gain5 : Gain  Gain=v_w_n
  Gain8 : Gain  Commented=through  Gain=omega_WTR_n
  Gain9 : Gain  Gain=omega_WTR_n
  Generator equations : Subsystem
  Pitch Controller : Subsystem
  Subsystem : Subsystem
  Sum1 : Sum  Inputs=|++
  Two mass module : Subsystem
  wind ramp : FromWorkspace  VariableName=wind_array
  Beta : Outport
  T_em : Outport  Port=2
  omega_gen : Outport  Port=3
  P MPPT : Outport  Port=4
  wires:
  [omega_gen] -> Gain2/1
  [omega_WTR] -> Subsystem/1(omega_wtr)  "omega_wtr"
  [i_d] -> Current control/2(i_d_meas)  "i_d_meas"
  Generator equations/3(Out3) -> [i_q]
  [i_q] -> Generator equations/5(i_q_meas)  "i_q_meas"
  Pitch Controller/1(Beta) -> Beta/1
  [i_d] -> Generator equations/4(i_d_meas)  "i_d_meas"
  Constant18/1 -> Aerodynamic power/1(R_WTR)
  [omega_gen] -> Generator equations/2(omega_elec)  "omega_elec"
  Gain5/1 -> Aerodynamic power/4(wind speed), [U]
  P ag/1 -> Two mass module/2(P ag)
  Constant11/1 -> Gain4/1
  wind ramp/1 -> ?
  [P_aero_cp] -> Two mass module/1(p_aero)
  Constant4/1 -> Current control/1(i_d_ref)  "i_d_ref"
  Generator equations/1(Out1) -> [Torque_em]
  Constant5/1 -> Sum1/2
  Two mass module/1(omega_WTR) -> [omega_WTR]
  [P_MPPT] -> Divide1/2
  Two mass module/2(omega_gen) -> [omega_gen]
  [omega_gen] -> Divide1/1, Current control/3(omega_elec)  "omega_elec"
  Sum1/1 -> Pitch Controller/2(ref)
  Gain4/1 -> Sum1/1, Display1/1  "omega_wtr"
  Constant6/1 -> Gain3/1
  [omega_WTR] -> Gain8/1
  Clock/1 -> 2-D Lookup Table/1
  Pitch Controller/2(Beta1) -> [Beta]
  [i_q] -> Current control/4(i_q_meas)  "i_q_meas"
  Aerodynamic power/1(P_aero) -> [P_aero_cp]
  Gain9/1 -> Aerodynamic power/3(omega_WTR)
  Gain8/1 -> Display2/1, Pitch Controller/1(meas)
  [Beta] -> Aerodynamic power/2(Theta)
  2-D Lookup Table/1 -> Gain5/1
  [Torque_em] -> Gain/1
  Subsystem/1(P MPPT) -> P MPPT/1, [P_MPPT]
  Divide1/1 -> Current control/5(torque_ref)  "torque_ref"
  Current control/1(v_d_ref) -> Generator equations/1(v_d_ref)
  Generator equations/2(Out2) -> [i_d]
  [omega_WTR] -> Gain9/1
  Current control/2(v_q_ref) -> Generator equations/3(v_q_ref)
  Gain/1 -> T_em/1
  Gain2/1 -> omega_gen/1

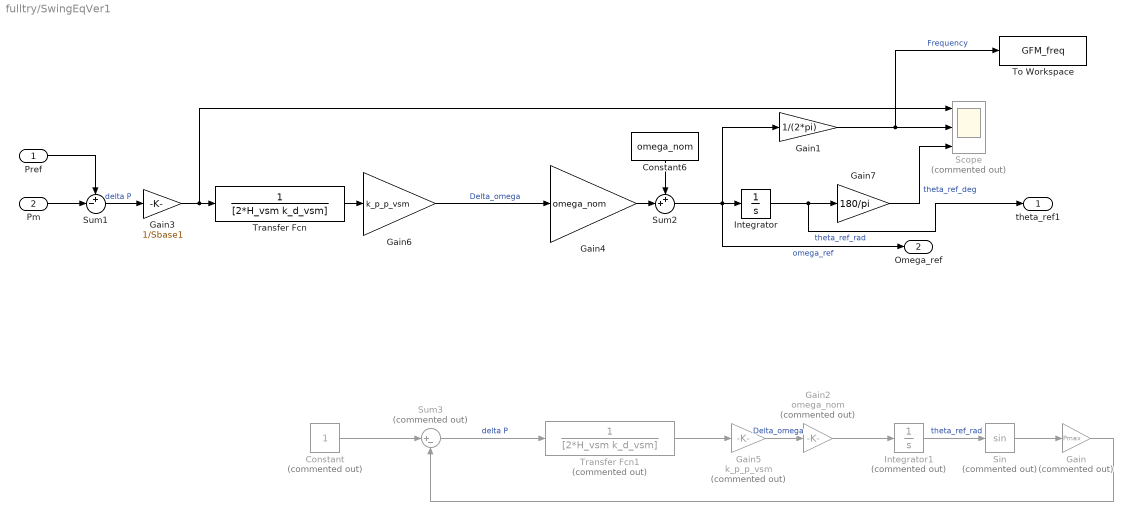
== system fulltry/SwingEqVer1 ==
  Pref : Inport
  Pm : Inport  Port=2
  Constant : Constant  Commented=on
  Constant6 : Constant  Value=omega_nom
  Gain : Gain  Commented=on  Gain=Pmax
  Gain1 : Gain  Gain=1/(2*pi)
  Gain2 : Gain  Commented=on  Gain=omega_nom
  Gain3 : Gain  Gain=1/Sbase1
  Gain4 : Gain  Gain=omega_nom
  Gain5 : Gain  Commented=on  Gain=k_p_p_vsm
  Gain6 : Gain  Gain=k_p_p_vsm
  Gain7 : Gain  Gain=180/pi
  Integrator : Integrator  WrappedStateUpperValue=2*pi  WrappedStateLowerValue=0
  Integrator1 : Integrator  Commented=on  WrappedStateUpperValue=2*pi  WrappedStateLowerValue=0
  Scope : Scope  Commented=on  NumInputPorts=3
  Sin : Trigonometry  Commented=on
  Sum1 : Sum  Inputs=+-|
  Sum2 : Sum  Inputs=++|
  Sum3 : Sum  Commented=on  Inputs=|+-
  To Workspace : ToWorkspace  VariableName=GFM_freq  SaveFormat=Structure With Time  SampleTime=-1
  Transfer Fcn : TransferFcn  Denominator=[2*H_vsm k_d_vsm]
  Transfer Fcn1 : TransferFcn  Commented=on  Denominator=[2*H_vsm k_d_vsm]
  theta_ref1 : Outport
  Omega_ref : Outport  Port=2
  wires:
  Sum1/1 -> Gain3/1  "delta P"
  Integrator/1 -> theta_ref1/1, Gain7/1  "theta_ref_rad"
  Sum2/1 -> Gain1/1, Omega_ref/1, Integrator/1  "omega_ref"
  Transfer Fcn/1 -> Gain6/1
  Gain6/1 -> Gain4/1  "Delta_omega"
  Pm/1 -> Sum1/2
  Gain3/1 -> Scope/1, Transfer Fcn/1
  Gain7/1 -> Scope/3  "theta_ref_deg"
  Pref/1 -> Sum1/1
  Constant6/1 -> Sum2/1
  Gain4/1 -> Sum2/2
  Gain1/1 -> To Workspace/1, Scope/2  "Frequency"
  Gain5/1 -> Gain2/1  "Delta_omega"
  Transfer Fcn1/1 -> Gain5/1
  Sum3/1 -> Transfer Fcn1/1  "delta P"
  Gain2/1 -> Integrator1/1
  Sin/1 -> Gain/1
  Gain/1 -> Sum3/2
  Constant/1 -> Sum3/1
  Integrator1/1 -> Sin/1  "theta_ref_rad"

== system fulltry/Voltage control ==
  Qm : Inport
  Qref : Inport  Port=2
  Constant5 : Constant
  Gain8 : Gain  Gain=1/Sbase1
  Gain9 : Gain  Gain=k_p_q_vsm
  Scope : Scope  NumInputPorts=5
  Sum3 : Sum  Inputs=|-+
  Sum4 : Sum  Inputs=|++
  Transfer Fcn1 : TransferFcn  Numerator=[ki_q]  Denominator=[1 ki_q]
  Vref : Outport
  delta Q : Outport  Port=2
  wires:
  Constant5/1 -> Sum4/2
  Qm/1 -> Sum3/1
  Gain9/1 -> Scope/4, Sum4/1
  Transfer Fcn1/1 -> Scope/3, Gain9/1
  Gain8/1 -> Scope/2, Transfer Fcn1/1
  Sum3/1 -> Scope/1, delta Q/1, Gain8/1  "delta Q"
  Sum4/1 -> Scope/5, Vref/1  "Vref"
  Qref/1 -> Sum3/2

== system fulltry/WT power ==
  I_dc : Inport
  Controlled Current Source : spsControlledCurrentSourceLib/Controlled Current Source  Initialize=on  Source_Type=DC  Amplitude=0  Phase=0  Frequency=0  Measurements=None
  Current Measurement1 : spsCurrentMeasurementLib/Current Measurement  PhasorSimulation=off  OutputType=Complex  PSBequivalent=0
  Product1 : Product  SaturateOnIntegerOverflow=on  OutDataTypeStr=Inherit: Same as first input
  Voltage Measurement1 : spsVoltageMeasurementLib/Voltage Measurement  PhasorSimulation=off  OutputType=Complex  PSBequivalent=0
  + : PMIOPort  Side=Right
  - : PMIOPort  Port=2  Side=Right
  Pwt : Outport
  V_dc_meas : Outport  Port=2
  i_dc_meas : Outport  Port=3
  wires:
  Current Measurement1/1 -> i_dc_meas/1, Product1/1
  Product1/1 -> Pwt/1
  Voltage Measurement1/1 -> V_dc_meas/1, Product1/2
  I_dc/1 -> Controlled Current Source/1
  connections:
  Controlled Current Source/LConn1 -- Voltage Measurement1/LConn2 -- -/RConn1
  Current Measurement1/LConn1 -- Voltage Measurement1/LConn1 -- +/RConn1
  Current Measurement1/RConn1 -- Controlled Current Source/RConn1

== system fulltry/constant DC Voltage ==
  DC Voltage Source2 : spsDCVoltageSourceLib/DC Voltage Source  Amplitude=V_dc/2  Measurements=None
  DC Voltage Source3 : spsDCVoltageSourceLib/DC Voltage Source  Amplitude=V_dc/2  Measurements=None
  + : PMIOPort  Side=Left
  - : PMIOPort  Port=2  Side=Right
  connections:
  DC Voltage Source2/LConn1 -- DC Voltage Source3/RConn1
  DC Voltage Source2/RConn1 -- +/RConn1
  DC Voltage Source3/LConn1 -- -/RConn1

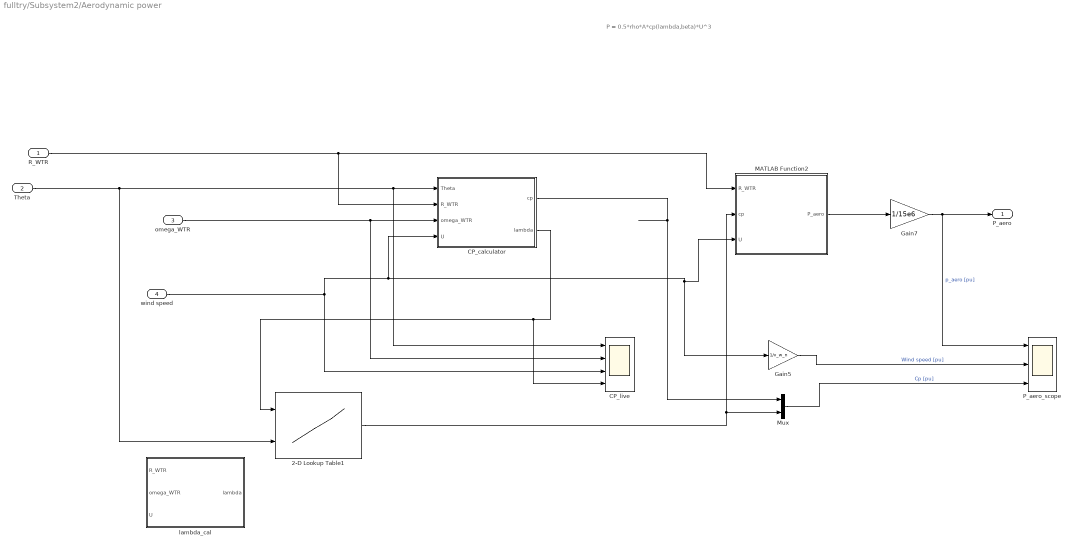
== system fulltry/Subsystem2/Aerodynamic power ==
  note: P = 0.5*rho*A*cp(lambda,beta)*U^3
  R_WTR : Inport
  Theta : Inport  Port=2
  omega_WTR : Inport  Port=3
  wind speed : Inport  Port=4
  2-D Lookup Table1 : Lookup_n-D  BreakpointsForDimension1=TSRvector  BreakpointsForDimension2=Pitchanglevector  Table=Powercoefficient  InternalRulePriority=Speed  RndMeth=Simplest
      settings: InputPortMap=u0,u1
  CP_calculator : MATLAB Function  TreatAsAtomicUnit=on
  CP_live : Scope  NumInputPorts=4
  Gain5 : Gain  Gain=1/v_w_n
  Gain7 : Gain  Gain=1/15e6
  MATLAB Function2 : MATLAB Function  TreatAsAtomicUnit=on
  Mux : Mux  Inputs=2
  P_aero_scope : Scope  NumInputPorts=3
  lambda_cal : MATLAB Function  TreatAsAtomicUnit=on
  P_aero : Outport
  wires:
  R_WTR/1 -> CP_calculator/2(R_WTR), MATLAB Function2/1(R_WTR)
  wind speed/1 -> Gain5/1, MATLAB Function2/3(U), CP_calculator/4(U), CP_live/3
  Theta/1 -> 2-D Lookup Table1/2, CP_live/1, CP_calculator/1(Theta)
  omega_WTR/1 -> CP_calculator/3(omega_WTR), CP_live/2
  MATLAB Function2/1(P_aero) -> Gain7/1
  CP_calculator/2(lambda) -> CP_live/4, 2-D Lookup Table1/1
  Gain7/1 -> P_aero_scope/1, P_aero/1  "p_aero [pu]"
  CP_calculator/1(cp) -> Mux/1
  Gain5/1 -> P_aero_scope/2  "Wind speed [pu]"
  2-D Lookup Table1/1 -> Mux/2, MATLAB Function2/2(cp)
  Mux/1 -> P_aero_scope/3  "Cp [pu]"

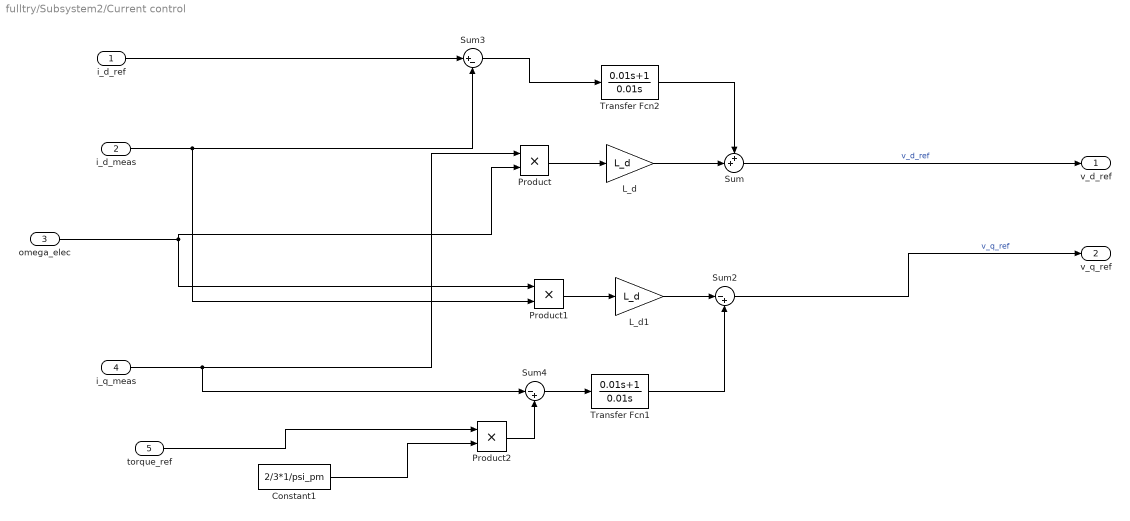
== system fulltry/Subsystem2/Current control ==
  i_d_ref : Inport
  i_d_meas : Inport  Port=2
  omega_elec : Inport  Port=3
  i_q_meas : Inport  Port=4
  torque_ref : Inport  Port=5
  Constant1 : Constant  Value=2/3*1/psi_pm
  L_d : Gain  Gain=L_d
  L_d1 : Gain  Gain=L_d
  Product : Product
  Product1 : Product
  Product2 : Product
  Sum : Sum  Inputs=++|
  Sum2 : Sum  Inputs=|-+
  Sum3 : Sum  Inputs=|+-
  Sum4 : Sum  Inputs=|-+
  Transfer Fcn1 : TransferFcn  Numerator=[0.01 1]  Denominator=[0.01 0]
  Transfer Fcn2 : TransferFcn  Numerator=[0.01 1]  Denominator=[0.01 0]
  v_d_ref : Outport
  v_q_ref : Outport  Port=2
  wires:
  Sum3/1 -> Transfer Fcn2/1
  L_d1/1 -> Sum2/1
  Transfer Fcn2/1 -> Sum/1
  omega_elec/1 -> Product/2, Product1/1
  Constant1/1 -> Product2/2
  Sum4/1 -> Transfer Fcn1/1
  Product2/1 -> Sum4/2
  Product/1 -> L_d/1
  Sum/1 -> v_d_ref/1  "v_d_ref"
  Transfer Fcn1/1 -> Sum2/2
  i_d_meas/1 -> Product1/2, Sum3/2
  Product1/1 -> L_d1/1
  L_d/1 -> Sum/2
  i_q_meas/1 -> Sum4/1, Product/1
  i_d_ref/1 -> Sum3/1
  torque_ref/1 -> Product2/1
  Sum2/1 -> v_q_ref/1  "v_q_ref"

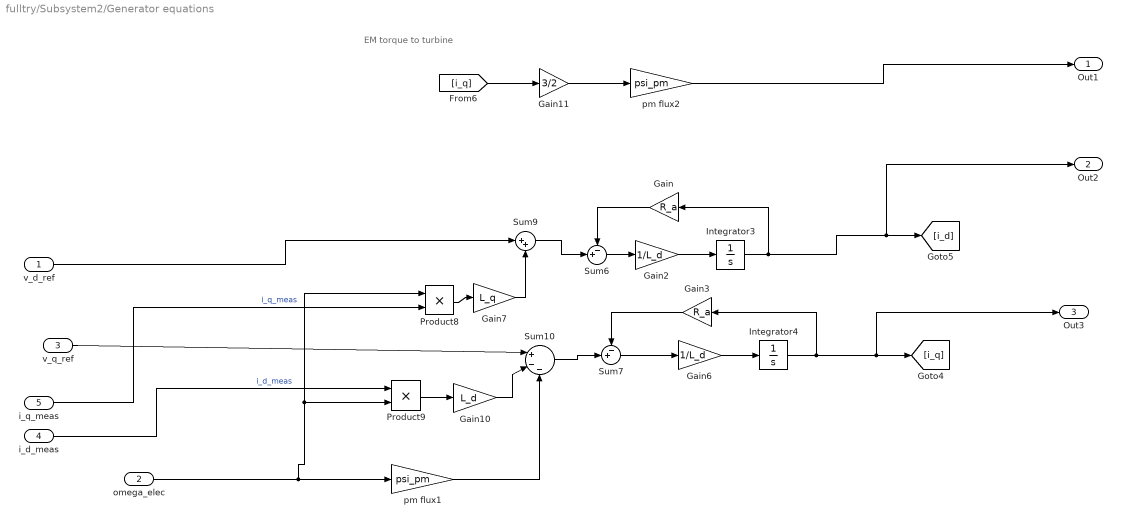
== system fulltry/Subsystem2/Generator equations ==
  note: EM torque to turbine
  v_d_ref : Inport
  omega_elec : Inport  Port=2
  v_q_ref : Inport  Port=3
  i_d_meas : Inport  Port=4
  i_q_meas : Inport  Port=5
  Gain : Gain  Gain=R_a
  Gain10 : Gain  Gain=L_d
  Gain11 : Gain  Gain=3/2
  Gain2 : Gain  Gain=1/L_d
  Gain3 : Gain  Gain=R_a
  Gain6 : Gain  Gain=1/L_d
  Gain7 : Gain  Gain=L_q
  Integrator3 : Integrator
  Integrator4 : Integrator  InitialCondition=2.3e4
  Product8 : Product
  Product9 : Product
  Sum10 : Sum  Inputs=|+--
  Sum6 : Sum  Inputs=-+|
  Sum7 : Sum  Inputs=-+|
  Sum9 : Sum  Inputs=|++
  pm flux1 : Gain  Gain=psi_pm
  pm flux2 : Gain  Gain=psi_pm
  Out1 : Outport
  Out2 : Outport  Port=2
  Out3 : Outport  Port=3
  wires:
  Gain6/1 -> Integrator4/1
  Integrator4/1 -> Out3/1, [i_q], Gain3/1
  Sum10/1 -> Sum7/2
  v_d_ref/1 -> Sum9/1
  Product8/1 -> Gain7/1
  Sum7/1 -> Gain6/1
  Gain2/1 -> Integrator3/1
  pm flux1/1 -> Sum10/3
  Sum9/1 -> Sum6/2
  omega_elec/1 -> Product8/1, Product9/2, pm flux1/1
  [i_q] -> Gain11/1
  Gain3/1 -> Sum7/1
  Gain11/1 -> pm flux2/1
  Sum6/1 -> Gain2/1
  Gain10/1 -> Sum10/2
  Gain/1 -> Sum6/1
  Integrator3/1 -> Gain/1, Out2/1, [i_d]
  Product9/1 -> Gain10/1
  i_q_meas/1 -> Product8/2  "i_q_meas"
  i_d_meas/1 -> Product9/1  "i_d_meas"
  Gain7/1 -> Sum9/2
  v_q_ref/1 -> Sum10/1
  pm flux2/1 -> Out1/1

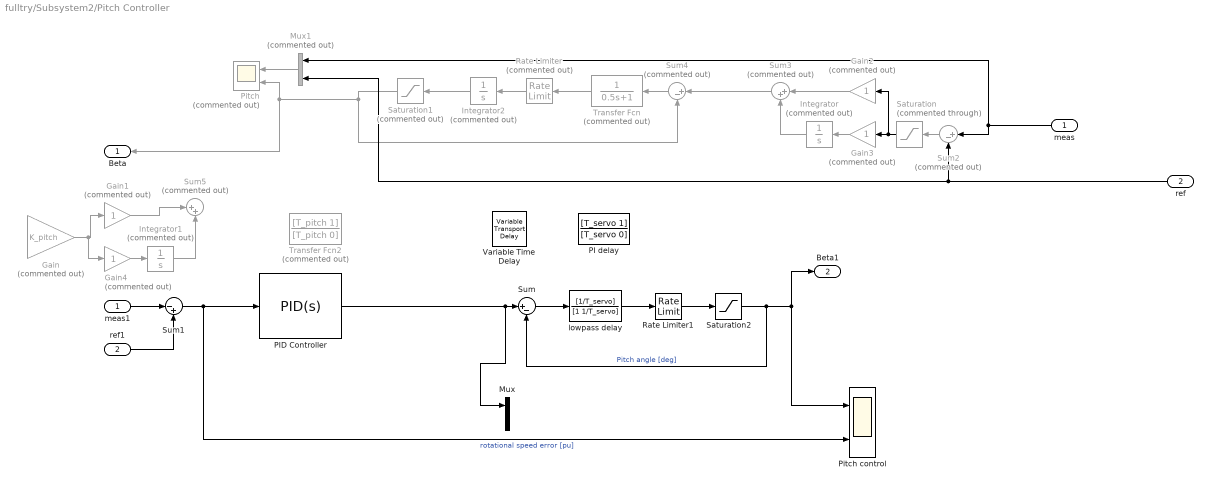
== system fulltry/Subsystem2/Pitch Controller ==
  meas : Inport
  ref : Inport  Port=2
  Gain : Gain  Commented=on  Gain=K_pitch
  Gain{1..4} (4 alike) : Gain  Commented=on
  Integrator : Integrator  Commented=on
  Integrator1 : Integrator  Commented=on  LimitOutput=on  UpperSaturationLimit=pitch_max  LowerSaturationLimit=pitch_min
  Integrator2 : Integrator  Commented=on
  Mux : Mux  Inputs=2
  Mux1 : Mux  Commented=on  Inputs=2
  PI delay : TransferFcn  Numerator=[T_servo 1]  Denominator=[T_servo 0]
  PID Controller : slpidlib/PID Controller  Controller=PID  Form=Ideal  TimeDomain=Continuous-time  UseExternalTs=off  SampleTime=-1  IntegratorMethod=Forward Euler  FilterMethod=Forward Euler  ControllerParametersSource=internal  P=K_pitch  I=T_pitch  UseKiTs=on  D=0  N=100  UseFilter=on  TunerSelectOption=Transfer Function Based (PID Tuner App)  InitialConditionSource=internal  InitialConditionForIntegrator=0  InitialConditionForFilter=0  DifferentiatorICPrevScaledInput=0  ExternalReset=none  TrackingMode=off  Kt=1  LimitOutput=on  SatLimitsSource=internal  UpperSaturationLimit=pitch_max  LowerSaturationLimit=pitch_min  LinearizeAsGain=on  AntiWindupMode=clamping  Kb=1  LimitIntegrator=off  UpperIntegratorSaturationLimit=inf  LowerIntegratorSaturationLimit=-inf  POutMin=[]  POutMax=[]  IOutMin=[]  IOutMax=[]  DOutMin=[]  DOutMax=[]  NOutMin=[]  NOutMax=[]  SumOutMin=[]  SumOutMax=[]  SaturationOutMin=[]  SaturationOutMax=[]  PParamMin=[]  PParamMax=[]  IParamMin=[]  IParamMax=[]  DParamMin=[]  DParamMax=[]  NParamMin=[]  NParamMax=[]  KbParamMin=[]  KbParamMax=[]  KtParamMin=[]  KtParamMax=[]  KbOutMin=[]  KbOutMax=[]  KtOutMin=[]  KtOutMax=[]  IntegratorOutMin=[]  IntegratorOutMax=[]  FilterOutMin=[]  FilterOutMax=[]  SumI1OutMin=[]  SumI1OutMax=[]  SumI2OutMin=[]  SumI2OutMax=[]  SumI3OutMin=[]  SumI3OutMax=[]  SumI4OutMin=[]  SumI4OutMax=[]  SumDOutMin=[]  SumDOutMax=[]  DifferentiatorOutMin=[]  DifferentiatorOutMax=[]  FilterDiffOutCoefMin=[]  FilterDiffOutCoefMax=[]  ReciprocalOutMin=[]  ReciprocalOutMax=[]  SumDenOutMin=[]  SumDenOutMax=[]  SumNumOutMin=[]  SumNumOutMax=[]  DivideOutMin=[]  DivideOutMax=[]  UdiffTsProdOutMin=[]  UdiffTsProdOutMax=[]  NTsProdOutMin=[]  NTsProdOutMax=[]  UintegralTsProdOutMin=[]  UintegralTsProdOutMax=[]  UngainTsProdOutMin=[]  UngainTsProdOutMax=[]  ClampingZeroOutDataTypeStr=Inherit: Inherit via back propagation  ClampingZeroOutMin=[]  ClampingZeroOutMax=[]  FilterDenConstantOutDataTypeStr=Inherit: Inherit via back propagation  FilterDenConstantOutMin=[]  FilterDenConstantOutMax=[]  PCopyOutDataTypeStr=Inherit: Inherit via back propagation  PCopyOutMin=[]  PCopyOutMax=[]  NCopyOutDataTypeStr=Inherit: Inherit via back propagation  NCopyOutMin=[]  NCopyOutMax=[]  IntegratorContinuousStateAttributes=''  IntegratorStateMustResolveToSignalObject=off  IntegratorRTWStateStorageClass=Auto  FilterContinuousStateAttributes=''  FilterStateMustResolveToSignalObject=off  FilterRTWStateStorageClass=Auto  ParallelPVariant=Passthrough  IdealPVariant=InternalParameters  IVariant=InternalParameters  DVariant=InternalParameters  IntegratorVariant=Continuous  SatVariant=Enabled  AWVariant=ContClampingIdeal  PCopyVariant=InternalParamsIdeal  TRVariant=Disabled  FdbkBlocksVariant=Forward  IdealPFdbkVariant=Disabled  SatFdbkVariant=Disabled  DerivativeFilterVariant=ContFilter  NVariant=InternalParameters  NCopyVariant=Disabled  FilterICVariant=InternalICsFilter  IntegratorICVariant=InternalICs  ExternalResetVariant=Disabled  TRSumVariant=Passthrough  SumFdbkVariant=Disabled  SumVariant=Sum_PID  TsampFilterVariant=InternalTs  TsampNgainVariant=Passthrough  TsampIntegralVariant=Disabled_SignalSpec  ExternalSaturationOutDataTypeStr=Inherit: Same as second input
  Pitch : Scope  Commented=on  NumInputPorts=2
  Pitch control : Scope  NumInputPorts=2
  Rate Limiter : RateLimiter  Commented=on  RisingSlewLimit=5  FallingSlewLimit=-5  SampleTimeMode=inherited
  Rate Limiter1 : RateLimiter  RisingSlewLimit=rate_max  FallingSlewLimit=rate_min  SampleTimeMode=inherited
  Saturation : Saturate  Commented=through  UpperLimit=inf  LowerLimit=0
  Saturation1 : Saturate  Commented=on  UpperLimit=90  LowerLimit=0
  Saturation2 : Saturate  UpperLimit=pitch_max  LowerLimit=pitch_min
  Sum : Sum  Inputs=|+-
  Sum1 : Sum  Inputs=|-+
  Sum2 : Sum  Commented=on  Inputs=|+-
  Sum3 : Sum  Commented=on  Inputs=|++
  Sum4 : Sum  Commented=on  Inputs=|+-
  Sum5 : Sum  Commented=on  Inputs=|++
  Transfer Fcn : TransferFcn  Commented=on  Denominator=[0.5 1]
  Transfer Fcn2 : TransferFcn  Commented=on  Numerator=[T_pitch 1]  Denominator=[T_pitch 0]
  Variable Time Delay : VariableTransportDelay  MaximumDelay=T_servo
  lowpass delay : TransferFcn  Numerator=[1/T_servo]  Denominator=[1 1/T_servo]
  meas1 : InportShadow
  ref1 : InportShadow  Port=2
  Beta : Outport
  Beta1 : Outport  Port=2
  wires:
  Transfer Fcn/1 -> Rate Limiter/1
  meas/1 -> Sum2/1, Mux1/1
  Mux1/1 -> Pitch/1
  Sum2/1 -> Saturation/1
  Sum3/1 -> Sum4/1
  Saturation/1 -> Gain2/1, Gain3/1
  Saturation1/1 -> Beta/1, Pitch/2, Sum4/2
  Gain3/1 -> Integrator/1
  Gain2/1 -> Sum3/1
  Sum4/1 -> Transfer Fcn/1
  Rate Limiter/1 -> Integrator2/1
  Integrator/1 -> Sum3/2
  ref/1 -> Mux1/2, Sum2/2
  Integrator2/1 -> Saturation1/1
  Rate Limiter1/1 -> Saturation2/1
  Sum/1 -> lowpass delay/1
  lowpass delay/1 -> Rate Limiter1/1
  Saturation2/1 -> Beta1/1, Pitch control/1, Sum/2  "Pitch angle [deg]"
  meas1/1 -> Sum1/1
  ref1/1 -> Sum1/2
  PID Controller/1 -> Mux/1, Sum/1
  Sum1/1 -> PID Controller/1, Pitch control/2  "rotational speed error [pu]"
  Gain4/1 -> Integrator1/1
  Gain1/1 -> Sum5/1
  Integrator1/1 -> Sum5/2
  Gain/1 -> Gain4/1, Gain1/1

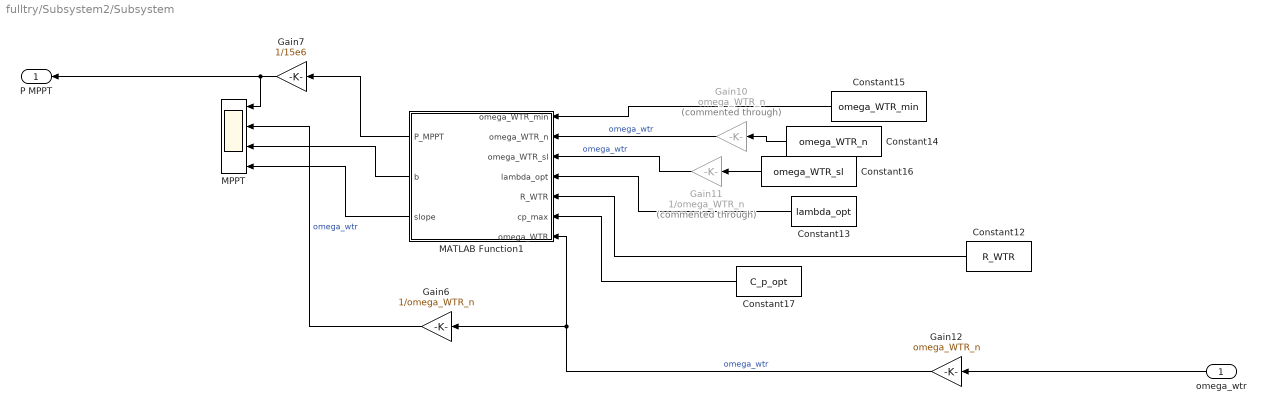
== system fulltry/Subsystem2/Subsystem ==
  omega_wtr : Inport
  Constant12 : Constant  Value=R_WTR
  Constant13 : Constant  Value=lambda_opt
  Constant14 : Constant  Value=omega_WTR_n
  Constant15 : Constant  Value=omega_WTR_min
  Constant16 : Constant  Value=omega_WTR_sl
  Constant17 : Constant  Value=C_p_opt
  Gain10 : Gain  Commented=through  Gain=omega_WTR_n
  Gain11 : Gain  Commented=through  Gain=1/omega_WTR_n
  Gain12 : Gain  Gain=omega_WTR_n
  Gain6 : Gain  Gain=1/omega_WTR_n
  Gain7 : Gain  Gain=1/15e6
  MATLAB Function1 : MATLAB Function  TreatAsAtomicUnit=on
  MPPT : Scope  NumInputPorts=4
  P MPPT : Outport
  wires:
  Constant17/1 -> MATLAB Function1/6(cp_max)
  MATLAB Function1/2(b) -> MPPT/3
  Constant13/1 -> MATLAB Function1/4(lambda_opt)
  Gain6/1 -> MPPT/2  "omega_wtr"
  Gain7/1 -> P MPPT/1, MPPT/1
  Gain12/1 -> MATLAB Function1/7(omega_WTR), Gain6/1  "omega_wtr"
  Gain11/1 -> MATLAB Function1/3(omega_WTR_sl)  "omega_wtr"
  MATLAB Function1/1(P_MPPT) -> Gain7/1
  Constant15/1 -> MATLAB Function1/1(omega_WTR_min)
  Gain10/1 -> MATLAB Function1/2(omega_WTR_n)  "omega_wtr"
  Constant14/1 -> Gain10/1
  Constant16/1 -> Gain11/1
  Constant12/1 -> MATLAB Function1/5(R_WTR)
  MATLAB Function1/3(slope) -> MPPT/4
  omega_wtr/1 -> Gain12/1

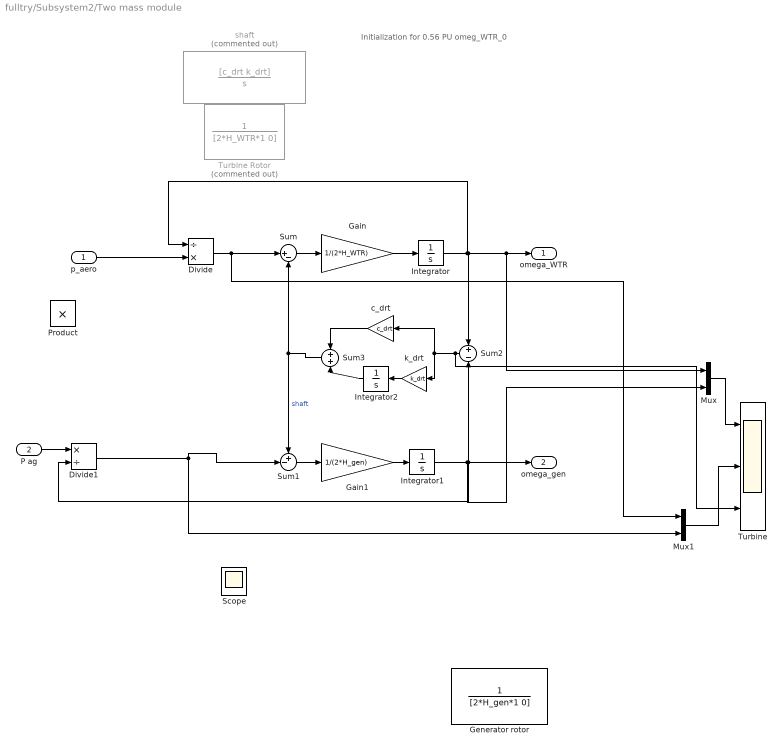
== system fulltry/Subsystem2/Two mass module ==
  note: Initialization for 0.56 PU omeg_WTR_0
  p_aero : Inport
  P ag : Inport  Port=2
  Divide : Product  Inputs=/*
  Divide1 : Product  Inputs=*/
  Gain : Gain  Gain=1/(2*H_WTR)
  Gain1 : Gain  Gain=1/(2*H_gen)
  Generator rotor : TransferFcn  Denominator=[2*H_gen*1 0]
  Integrator : Integrator  InitialCondition=omega_WTR_min/omega_WTR_n
  Integrator1 : Integrator  InitialCondition=omega_WTR_min/omega_WTR_n
  Integrator2 : Integrator
  Mux : Mux  Inputs=2
  Mux1 : Mux  Inputs=2
  Product : Product
  Scope : Scope  NumInputPorts=2
  Sum : Sum  Inputs=|+-
  Sum1 : Sum  Inputs=+-|
  Sum2 : Sum  Inputs=+|-
  Sum3 : Sum  Inputs=+|+
  Turbine : Scope  NumInputPorts=3
  Turbine Rotor : TransferFcn  Commented=on  Denominator=[2*H_WTR*1 0]
  c_drt : Gain  Gain=c_drt
  k_drt : Gain  Gain=k_drt
  shaft : TransferFcn  Commented=on  Numerator=[c_drt k_drt]  Denominator=[1 0]
  omega_WTR : Outport
  omega_gen : Outport  Port=2
  wires:
  Divide1/1 -> Mux1/2, Sum1/2
  Integrator1/1 -> Divide1/2, omega_gen/1, Sum2/2, Mux/2
  Sum3/1 -> Sum1/1, Sum/2  "shaft"
  Integrator/1 -> Divide/1, Mux/1, omega_WTR/1, Sum2/1
  Sum/1 -> Gain/1
  p_aero/1 -> Divide/2
  Gain/1 -> Integrator/1
  Gain1/1 -> Integrator1/1
  Sum1/1 -> Gain1/1
  Integrator2/1 -> Sum3/2
  c_drt/1 -> Sum3/1
  Sum2/1 -> Turbine/3, k_drt/1, c_drt/1
  k_drt/1 -> Integrator2/1
  Mux/1 -> Turbine/1
  Divide/1 -> Mux1/1, Sum/1
  P ag/1 -> Divide1/1
  Mux1/1 -> Turbine/2

== matlab function fulltry/Subsystem2/Aerodynamic power/lambda_cal ==
  data: R_WTR input; omega_WTR input; U input; lambda output
function lambda  = fcn(R_WTR,omega_WTR,U) 
    
    lambda = omega_WTR*R_WTR/U;

== matlab function fulltry/Subsystem2/Subsystem/MATLAB Function1 ==
  data: omega_WTR_min input; P_MPPT output; omega_WTR_n input; omega_WTR_sl input; lambda_opt input; R_WTR input; cp_max input; omega_WTR input; b output; slope output
function [P_MPPT,b,slope] = fcn(omega_WTR_min,omega_WTR_n,omega_WTR_sl,lambda_opt,R_WTR,cp_max,omega_WTR)

rho = 1.2225;
P_mppt_sl = 0.5*pi*rho*R_WTR^5*cp_max/lambda_opt^3*omega_WTR_sl^3; %
P_mppt_max = 0.5*pi*rho*R_WTR^5*cp_max/lambda_opt^3*omega_WTR_n^3;
slope = (P_mppt_max-P_mppt_sl)/(omega_WTR_n-omega_WTR_sl);
b = P_mppt_max-slope*omega_WTR_n;

if omega_WTR < omega_WTR_min*0.5
    y = 0;
elseif omega_WTR < omega_WTR_sl
    y = 0.5*pi*rho*R_WTR^5*cp_max/lambda_opt^3*omega_WTR^3;
elseif omega_WTR < omega_WTR_n % at 1.0236 pu the turbine reaches P = 15 MW 
    y  =slope*omega_WTR+b;
% 0.5*pi*rho*R_WTR^5*cp_zero_deg/lambda_not_opt^3*omega_WTR^3;
else
    y = 15e6;%0.5*pi*rho*R_WTR^5*cp_max/lambda_opt^3*(omega_WTR_n)^3;
    
end

P_MPPT = y ;

== matlab function fulltry/Subsystem2/Aerodynamic power/MATLAB Function2 ==
  data: R_WTR input; cp input; P_aero output; U input
function P_aero = fcn(R_WTR,cp,U)

rho = 1.225;
P_aero = 0.5*pi*rho*R_WTR^2*cp*U^3;
